simulink model "beats"  (Simulink 10.1)
settings: Solver=VariableStepDiscrete  StartTime=0.0  StopTime=10  RelTol=1e-3  EnableMultiTasking=on
libraries: speaker x1
settings Model: Creator=Administrator  LastModifiedBy=elezhan
settings DataIOCC: LimitDataPoints=on  SignalLoggingSaveFormat=ModelDataLogs
settings OptimizationCC: ExpressionDepthLimit=2147483647
settings DebuggingCC: SolverPrmCheckMsg=warning  FcnCallInpInsideContextMsg=warning  StateNameClashWarn=warning

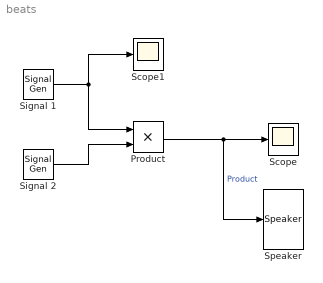
== system beats ==
  Product : Product  RndMeth=Zero
  Scope : Scope
  Scope1 : Scope
  Signal 1 : SignalGenerator  Frequency=400
  Signal 2 : SignalGenerator  Frequency=1/5
  Speaker : speaker/Speaker
  wires:
  Signal 1/1 -> Product/1, Scope1/1
  Signal 2/1 -> Product/2
  Product/1 -> Speaker/1, Scope/1  "Product"
